simulink model "LoopShaping_test"  (R2018a)
settings: Solver=VariableStepAuto  StartTime=0.0  StopTime=10  RelTol=1e-3  EnableMultiTasking=on
values from neighbouring files (symbols this model uses):
  Dg = cell2mat(G.den)    [LoopShaping_m.m]
  Dk = cell2mat(tf(K1).den)    [LoopShaping_m.m]
  Dk2 = cell2mat(tf(K2).den)    [LoopShaping_m.m]
  Ng = cell2mat(G.num)    [LoopShaping_m.m]
  Nk = cell2mat(tf(K1).num)    [LoopShaping_m.m]
  Nk2 = cell2mat(tf(K2).num)    [LoopShaping_m.m]
libraries: simulink x2
settings Model: Creator=user  LastModifiedBy=htngo2018
settings DataIOCC: LimitDataPoints=on
settings OptimizationCC: LifeSpan=inf
settings DebuggingCC: AllowSymbolicDim=off  SFUnexpectedBacktrackingDiag=warning  SFNoUnconditionalDefaultTransitionDiag=warning  SFExecutionAtInitializationDiag=none
settings ModelReferenceCC: PropagateSignalLabelsOutOfModel=off
settings CodeAppCC: StateflowObjectComments=on
settings GRTTargetCC: TargetLangStandard=C89/C90 (ANSI)
settings ConfigComp: CovMetricSettings=dw  CovHtmlReporting=on  CovSaveCumulativeToWorkspaceVar=on  CovSaveSingleToWorkspaceVar=on  CovExternalEMLEnable=off

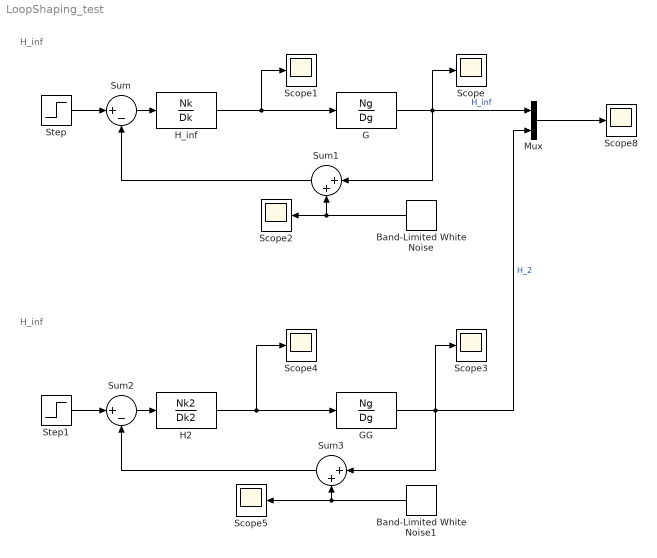
== system LoopShaping_test ==
  note: H_inf
  note: H_inf
  Band-Limited White Noise : simulink/Sources/Band-Limited White Noise  Cov=[1e-8]  Ts=1e-3  seed=[23341]
  Band-Limited White Noise1 : simulink/Sources/Band-Limited White Noise  Cov=[1e-8]  Ts=1e-3  seed=[23341]
  G : TransferFcn  Numerator=Ng  Denominator=Dg
  GG : TransferFcn  Numerator=Ng  Denominator=Dg
  H2 : TransferFcn  Numerator=Nk2  Denominator=Dk2
  H_inf : TransferFcn  Numerator=Nk  Denominator=Dk
  Mux : Mux  Inputs=2
  Scope{,1..5,8} (7 alike) : Scope
  Step : Step  SampleTime=0
  Step1 : Step  SampleTime=0
  Sum : Sum  Inputs=|+-
  Sum1 : Sum  Inputs=|++
  Sum2 : Sum  Inputs=|+-
  Sum3 : Sum  Inputs=|++
  wires:
  Sum/1 -> H_inf/1
  Step/1 -> Sum/1
  G/1 -> Mux/1, Scope/1, Sum1/1  "H_inf"
  Band-Limited White Noise/1 -> Scope2/1, Sum1/2
  Sum1/1 -> Sum/2
  Sum2/1 -> H2/1
  Step1/1 -> Sum2/1
  GG/1 -> Mux/2, Sum3/1, Scope3/1  "H_2"
  H2/1 -> GG/1, Scope4/1
  Band-Limited White Noise1/1 -> Scope5/1, Sum3/2
  Sum3/1 -> Sum2/2
  H_inf/1 -> G/1, Scope1/1
  Mux/1 -> Scope8/1
